simulink model "Duct_TestBed"  (R2012b)
settings: Solver=FixedStepDiscrete  StartTime=0.0  StopTime=1  FixedStep=1  RelTol=1e-3
undefined symbols (not defined in the file): MWS
libraries: Lib_Turbo_Duct_TMATS x1
settings Model: Creator=jwchapm2  LastModifiedBy=jwchapm2

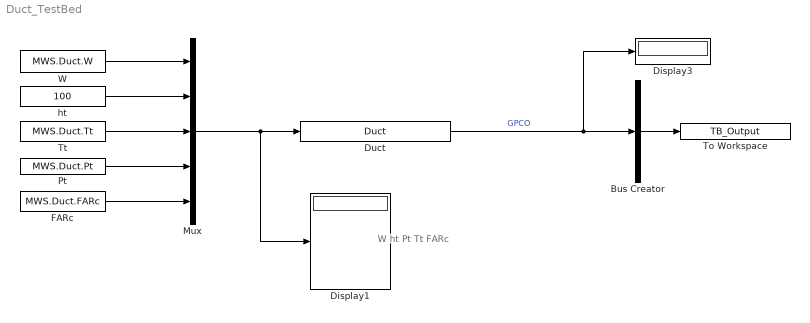
== system Duct_TestBed ==
  note: W
      | ht
      | Pt
      | Tt
      | FARc
  Bus Creator : BusCreator  Inputs=1
  Display1 : Display
  Display3 : Display
  Duct : Lib_Turbo_Duct_TMATS/Duct  dP_M=MWS.Duct.dP
  FARc : Constant  Value=MWS.Duct.FARc
  Mux : Mux  Inputs=5
  Pt : Constant  Value=MWS.Duct.Pt
  To Workspace : ToWorkspace  VariableName=TB_Output  SampleTime=-1
  Tt : Constant  Value=MWS.Duct.Tt
  W : Constant  Value=MWS.Duct.W
  ht : Constant  Value=100
  wires:
  W/1 -> Mux/1
  FARc/1 -> Mux/5
  Tt/1 -> Mux/3
  Pt/1 -> Mux/4
  Mux/1 -> Duct/1, Display1/1
  Duct/1 -> Display3/1, Bus Creator/1  "GPCO"
  Bus Creator/1 -> To Workspace/1
  ht/1 -> Mux/2
